simulink model "MicromouseMotor"  (R2023b)
settings: Solver=VariableStepAuto  StartTime=0.0  StopTime=1  RelTol=1e-3
settings Model: Creator=westj  LastModifiedBy=westj

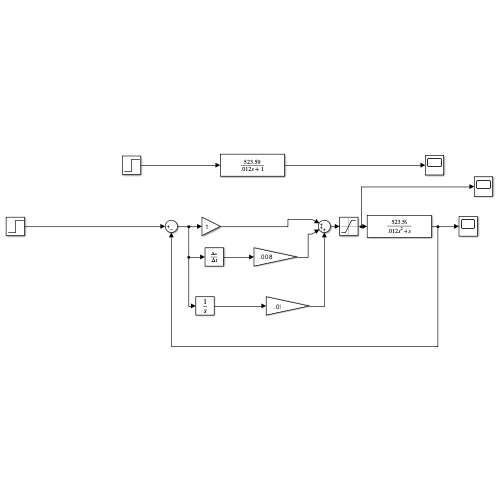
[thumbnail: Simulink's stored preview of the top-level diagram]
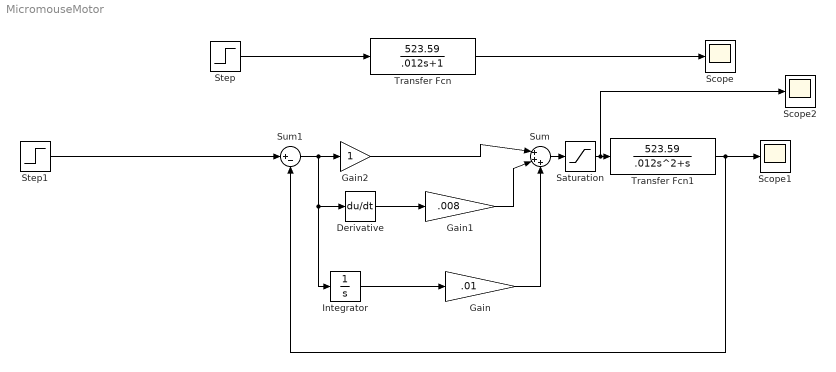
== system MicromouseMotor ==
  Derivative : Derivative
  Gain : Gain  Gain=.01
  Gain1 : Gain  Gain=.008
  Gain2 : Gain
  Integrator : Integrator
  Saturation : Saturate  UpperLimit=255  LowerLimit=-255
  Scope : Scope
  Scope1 : Scope
  Scope2 : Scope
  Step : Step  Time=.0001  SampleTime=.0001
  Step1 : Step  Time=.000001  After=10000  SampleTime=.001
  Sum : Sum  Inputs=|+++
  Sum1 : Sum  Inputs=|+-
  Transfer Fcn : TransferFcn  Numerator=[523.59]  Denominator=[.012 1]
  Transfer Fcn1 : TransferFcn  Numerator=[523.59]  Denominator=[.012 1 0]
  wires:
  Step/1 -> Transfer Fcn/1
  Transfer Fcn/1 -> Scope/1
  Integrator/1 -> Gain/1
  Derivative/1 -> Gain1/1
  Step1/1 -> Sum1/1
  Sum1/1 -> Integrator/1, Derivative/1, Gain2/1
  Gain2/1 -> Sum/1
  Gain1/1 -> Sum/2
  Gain/1 -> Sum/3
  Transfer Fcn1/1 -> Scope1/1, Sum1/2
  Sum/1 -> Saturation/1
  Saturation/1 -> Scope2/1, Transfer Fcn1/1
